simulink model "state_flow_chart"  (R2018b)
settings: Solver=VariableStepAuto  StartTime=0.0  StopTime=10.0  RelTol=1e-3
libraries: simulink x1
settings Model: Creator=marwan  LastModifiedBy=marwan

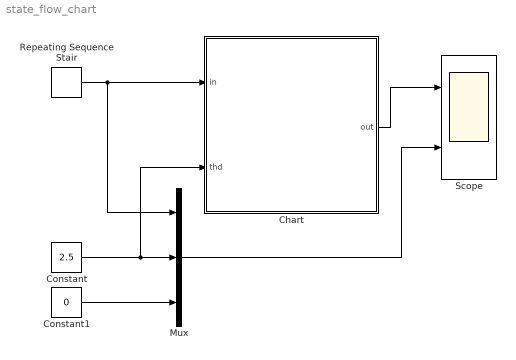
== system state_flow_chart ==
  Chart : Stateflow chart  TreatAsAtomicUnit=on
  Constant : Constant  Value=2.5
  Constant1 : Constant  Value=0
  Mux : Mux  Inputs=3
  Repeating Sequence Stair : simulink/Sources/Repeating Sequence Stair  OutValues=[3 0.5 1 -2 3 -2].'  tsamp=-1  OutMin=[]  OutMax=[]  OutDataTypeStr=double  OutputDataTypeScalingMode=double  OutDataType=fixdt(0,8)  ConRadixGroup=Best Precision: Vector-wise  OutScaling=2^-12
  Scope : Scope  NumInputPorts=2
  wires:
  Repeating Sequence Stair/1 -> Chart/1(in), Mux/1
  Constant/1 -> Chart/2(thd), Mux/2
  Constant1/1 -> Mux/3
  Mux/1 -> Scope/2
  Chart/1(out) -> Scope/1

== stateflow chart state_flow_chart/Chart ==
  (default) -> (junction 47) : % sys compare
  (junction 47) -> (junction 48) [order 1] : [in>thd]
  (junction 47) -> (junction 49) [order 2]
  (junction 48) -> (junction 53) : {out=1;}
  (junction 49) -> (junction 50) [order 1] : [in<=thd && in>0]
  (junction 49) -> (junction 51) [order 2] : {out=-1;}
  (junction 50) -> (junction 52) : {out=0;}
  (junction 52) -> (junction 51)
  (junction 53) -> (junction 52)
  (junction 51) -> (junction 54)
  data: in input; out output; thd input
